simulink model "PNG_radomeloop"  (R2019b)
settings: Solver=VariableStepAuto  StartTime=0.0  StopTime=10.0  FixedStep=0.01  RelTol=1e-3
settings Model: Creator=win10  LastModifiedBy=win10

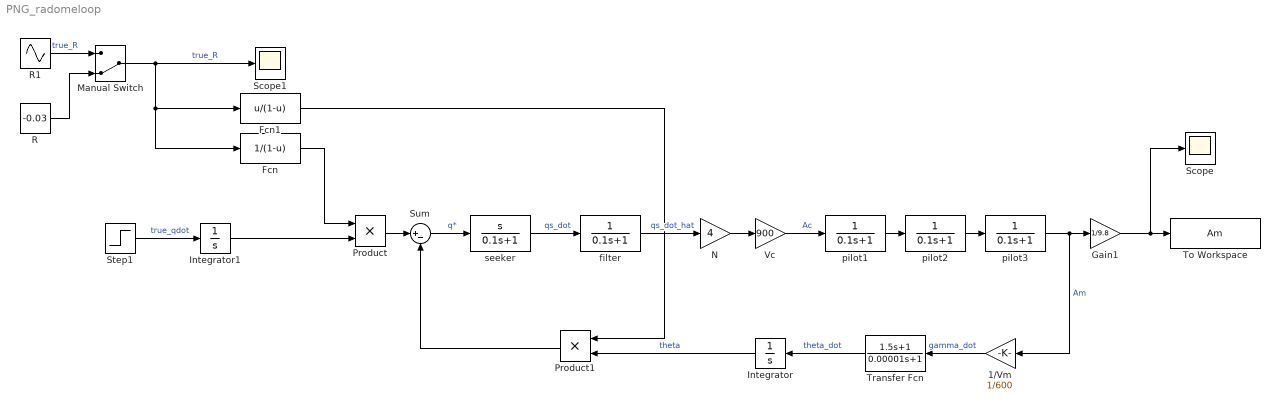
== system PNG_radomeloop ==
  1/Vm : Gain  Gain=1/600
  Fcn : Fcn  Expr=1/(1-u)
  Fcn1 : Fcn  Expr=u/(1-u)
  Gain1 : Gain  Gain=1/9.8
  Integrator : Integrator
  Integrator1 : Integrator
  Manual Switch : ManualSwitch  CurrentSetting=0
  N : Gain  Gain=4
  Product : Product
  Product1 : Product
  R : Constant  Value=-0.03
  R1 : Sin  Amplitude=0.06  Frequency=pi/2  SampleTime=0
  Scope : Scope
  Scope1 : Scope
  Step1 : Step  Time=0  After=pi/180  SampleTime=0
  Sum : Sum  Inputs=|+-
  To Workspace : ToWorkspace  VariableName=Am  SampleTime=-1
  Transfer Fcn : TransferFcn  Numerator=[1.5 1]  Denominator=[0.00001 1]
  Vc : Gain  Gain=900
  filter : TransferFcn  Denominator=[0.1 1]
  pilot1 : TransferFcn  Denominator=[0.1 1]
  pilot2 : TransferFcn  Denominator=[0.1 1]
  pilot3 : TransferFcn  Denominator=[0.1 1]
  seeker : TransferFcn  Numerator=[1 0]  Denominator=[0.1 1]
  wires:
  R1/1 -> Manual Switch/1  "true_R"
  R/1 -> Manual Switch/2
  Manual Switch/1 -> Scope1/1, Fcn1/1, Fcn/1  "true_R"
  Product/1 -> Sum/1
  Sum/1 -> seeker/1  "q*"
  seeker/1 -> filter/1  "qs_dot"
  filter/1 -> N/1  "qs_dot_hat"
  N/1 -> Vc/1
  Vc/1 -> pilot1/1  "Ac"
  pilot1/1 -> pilot2/1
  pilot2/1 -> pilot3/1
  1/Vm/1 -> Transfer Fcn/1  "gamma_dot"
  pilot3/1 -> Gain1/1, 1/Vm/1  "Am"
  Transfer Fcn/1 -> Integrator/1  "theta_dot"
  Integrator/1 -> Product1/2  "theta"
  Product1/1 -> Sum/2
  Step1/1 -> Integrator1/1  "true_qdot"
  Integrator1/1 -> Product/2
  Fcn/1 -> Product/1
  Fcn1/1 -> Product1/1
  Gain1/1 -> Scope/1, To Workspace/1
